simulink model "Target_Sim"  (R2025b)
settings: Solver=FixedStepAuto  StartTime=0.0  StopTime=10.0  RelTol=1e-3
undefined symbols (not defined in the file): t_rotation, t_size
settings Model: DataDictionary=Target_Sim_data.sldd  Creator=mauro  LastModifiedBy=mauro

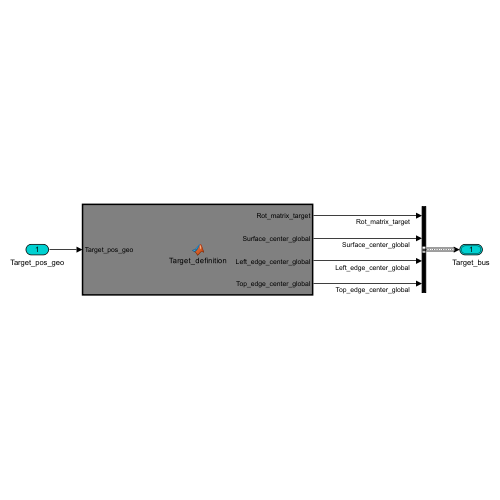
[thumbnail: Simulink's stored preview of the top-level diagram]
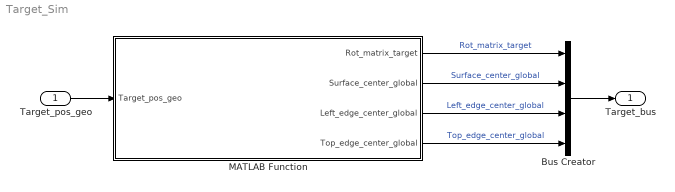
== system Target_Sim ==
  Target_pos_geo : Inport  PortDimensions=[3 1]
  Bus Creator : BusCreator  Inputs=4  OutDataTypeStr=Bus: Target_bus  NonVirtualBus=on
  MATLAB Function : MATLAB Function  TreatAsAtomicUnit=on
  Target_bus : Outport  OutDataTypeStr=Bus: Target_bus  BusOutputAsStruct=on
  wires:
  Target_pos_geo/1 -> MATLAB Function/1(Target_pos_geo)
  MATLAB Function/1(Rot_matrix_target) -> Bus Creator/1  "Rot_matrix_target"
  MATLAB Function/2(Surface_center_global) -> Bus Creator/2  "Surface_center_global"
  MATLAB Function/3(Left_edge_center_global) -> Bus Creator/3  "Left_edge_center_global"
  MATLAB Function/4(Top_edge_center_global) -> Bus Creator/4  "Top_edge_center_global"
  Bus Creator/1 -> Target_bus/1

== matlab function Target_Sim/MATLAB Function ==
  data: Rot_matrix_target output; Target_pos_geo input; Surface_center_global output; t_size parameter; t_rotation parameter; Left_edge_center_global output; Top_edge_center_global output
function [Rot_matrix_target,Surface_center_global,Left_edge_center_global,Top_edge_center_global] = Target_definition(Target_pos_geo,t_size, t_rotation)

Surface_center      = zeros(3,6);
Left_edge_center    = zeros(3,6);
Top_edge_center     = zeros(3,6);

Surface_center(:,1) = [-t_size(1)/2;0;0];% First Column, Surface code number 1: Face perpendicular to X axis, smaller (or more negative) X distance. Local reference system.
Surface_center(:,2) = [+t_size(1)/2;0;0];% Second Column, Surface code number 2: Face perpendicular to X axis, bigger (or less negative) X distance. Local reference system.
Surface_center(:,3) = [0;-t_size(2)/2;0];% Third Column, Surface code number 3: Face perpendicular to Y axis, smaller (or more negative) Y distance. Local reference system.
Surface_center(:,4) = [0;+t_size(2)/2;0];% Fourth Column, Surface code number 4: Face perpendicular to Y axis, bigger (or less negative) Y distance. Local reference system.
Surface_center(:,5) = [0;0;-t_size(3)/2];% Fifth Column, Surface code number 5: Face perpendicular to Z axis, smaller (or more negative) Z distance. Local reference system.
Surface_center(:,6) = [0;0;+t_size(3)/2];% Sixth Column, Surface code number 6: Face perpendicular to Z axis, bigger (or less negative) Z distance. Local reference system.

Left_edge_center(:,1) = [-t_size(1)/2;+t_size(2)/2;0];
Left_edge_center(:,2) = [+t_size(1)/2;-t_size(2)/2;0];
Left_edge_center(:,3) = [-t_size(1)/2;-t_size(2)/2;0];
Left_edge_center(:,4) = [+t_size(1)/2;+t_size(2)/2;0];
Left_edge_center(:,5) = [0;-t_size(2)/2;-t_size(3)/2];
Left_edge_center(:,6) = [0;+t_size(2)/2;+t_size(3)/2];

Top_edge_center(:,1) = [-t_size(1)/2;0;+t_size(3)/2];
Top_edge_center(:,2) = [+t_size(1)/2;0;+t_size(3)/2];
Top_edge_center(:,3) = [0;-t_size(2)/2;+t_size(3)/2];
Top_edge_center(:,4) = [0;+t_size(2)/2;+t_size(3)/2];
Top_edge_center(:,5) = [-t_size(1)/2;0;-t_size(3)/2];
Top_edge_center(:,6) = [-t_size(1)/2;0;+t_size(3)/2];

Surface_center_global   = zeros(3,6);
Left_edge_center_global = zeros(3,6);
Top_edge_center_global  = zeros(3,6);
Rot_matrix_target       = [sin(t_rotation) cos(t_rotation) 0;...
                           -cos(t_rotation) sin(t_rotation) 0;... 
                           0 0 1];

for i=1:length(Surface_center)

    Surface_center_global(:,i)    = Target_pos_geo+Rot_matrix_target*Surface_center(:,i)+[0;0;t_size(3)/2];
    Left_edge_center_global(:,i)  = Target_pos_geo+Rot_matrix_target*Left_edge_center(:,i)+[0;0;t_size(3)/2];
    Top_edge_center_global(:,i)   = Target_pos_geo+Rot_matrix_target*Top_edge_center(:,i)+[0;0;t_size(3)/2];

end
